simulink model "electrolyser_v4"  (R2022a)
settings: Solver=VariableStepAuto  StartTime=0.0  StopTime=10.0  RelTol=1e-3
model workspace: external: MATLAB File parameters_SS.m (data not in the file)
undefined symbols (not defined in the file or in its folder): clnt, const, input, pemel
libraries: fl_lib x24, nesl_utility x6, SimscapeFluids_lib x3
(part 2 of 2)

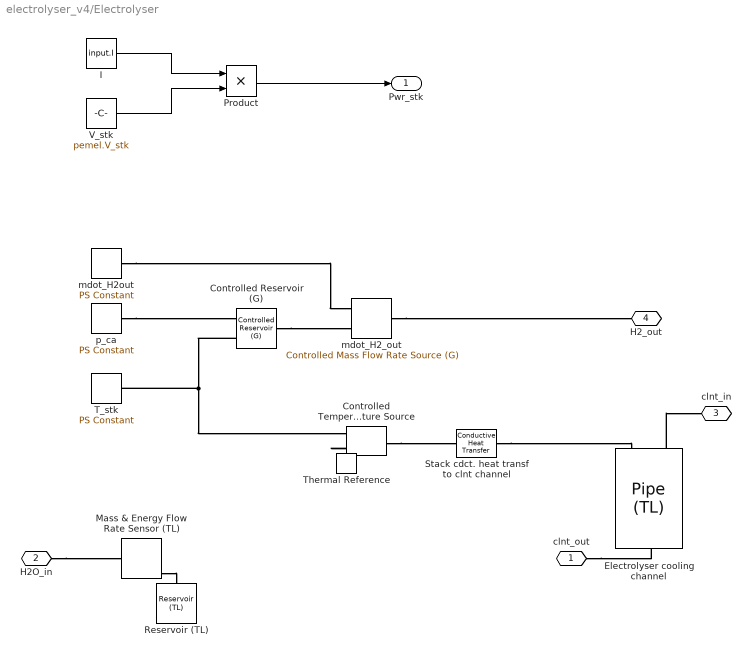
== system electrolyser_v4/Electrolyser ==
  Controlled Temperature Source : fl_lib/Thermal/Thermal Sources/Controlled Temperature Source
      settings: SourceProductBaseCode=PW,SS,VE
  Controlled Reservoir (G) : fl_lib/Gas/Elements/Controlled Reservoir (G)  area_A=pemel.totAc_ch_stk m^2
      settings: SourceProductBaseCode=PW,SS,VE  InternalSimscapePortConfiguration="{\"Bottom\":[],\"Left\":[{\"id\":\"A\",\"label\":\"A\",\"type\":\"foundation.gas.gas\"}],\"Right\":[{\"id\":\"T_in\",\"label\":\"T\",\"type\":\"input\"},{\"id\":\"p_in\",\"label\":\"P\",\"type\":\"input\"}],\"Top\":[]}"
  Electrolyser cooling channel : SimscapeFluids_lib/Thermal Liquid/Pipes & Fittings/Pipe (TL)  dynamic_compressibility=simscape.enum.onoff.off  inertia=simscape.enum.onoff.off  num_segments=1  pipe_length=pemel.L_clt m  area=pemel.totAc_clt_stk m^2  wall_spec=fluids.thermal_liquid.pipes_fittings.enum.wall_spec.rigid  Dh=pemel.Dh_clt m  wall_compliance=1.2e-6 m/MPa  wall_time_constant=0.01 s  elevation_spec=foundation.enum.constant_variable.constant  elevation_gain=0 m  g=9.81 m/s^2  pressure_loss_spec=fluids.thermal_liquid.pipes_fittings.enum.PressureLossSpec.Nominal  local_pressure_loss_spec=fluids.thermal_liquid.pipes_fittings.enum.LocalLossSpec.AggregateLength  length_add=1 m  loss_coefficient=0.1  roughness=15e-6 m  Re_friction_TLU=[400, 1000, 1500, 3000, 4000, 6000, 10000, 20000, 40000, 60000, 100000, 100000000]  friction_factor_TLU=[.264, .112, .071, .0417, .0387, .0268, .025, .0232, .0226, .022, .0214, .0214]  shape_factor=64  Re_lam=100000000  Re_tur=100000001  mdot_nominal=clnt.mdot_stk kg/s  p_diff_nominal=clnt.dp_stk Pa  mdot_threshold=1e-12 kg/s  heat_transfer_spec=fluids.thermal_liquid.pipes_fittings.enum.HeatTransferSpec.Nominal  mdot_nominal_heat=clnt.mdot_stk kg/s  T_in_nominal=clnt.T_stk_in K  T_out_nominal=clnt.T_stk_in + clnt.dT_stk K  p_in_nominal_heat=clnt.p_stk_in Pa  T_wall_nominal=pemel.T_stk K  a_coeff=0.023  b_Re_power=0.8  c_Pr_power=0.4  Nu_lam=3.66  Re_Colburn_TLU=[100, 150, 1000]  Colburn_factor_TLU=[.019, .013, .002]  Re_Nu_TLU=[100, 150, 1000]  Pr_Nu_TLU=[1, 10]  Nu_TLU=[3.72, 4.21; 3.75, 4.44; 4.21, 7.15]  T0_vec=amb.T K  p0_vec=0.101325 MPa  mdot0=0.1 kg/s
      settings: SourceProductBaseCode=SH
  I : Constant  Value=input.I
  Mass & Energy Flow Rate Sensor (TL) : fl_lib/Thermal Liquid/Sensors/Mass & Energy Flow Rate Sensor (TL)
      settings: SourceProductBaseCode=PW,SS,VE  InternalSimscapePortConfiguration="{\"Bottom\":[],\"Left\":[{\"id\":\"A\",\"label\":\"A\",\"type\":\"foundation.thermal_liquid.thermal_liquid\"}],\"Right\":[{\"id\":\"B\",\"label\":\"B\",\"type\":\"foundation.thermal_liquid.thermal_liquid\"},{\"id\":\"M\",\"label\":\"M\",\"type\":\"output\"},{\"id\":\"PHI\",\"label\":\"Phi\",\"type\":\"output\"}],\"Top\":[]}"
  Product : Product
  Reservoir (TL) : fl_lib/Thermal Liquid/Elements/Reservoir (TL)  pressure_spec=foundation.enum.pressure_spec.atmospheric  reservoir_pressure=0.101325 MPa  reservoir_temperature=293.15 K  area=pemel.totAc_ch_stk m^2
      settings: SourceProductBaseCode=PW,SS,VE
  Stack cdct. heat transf to clnt channel : fl_lib/Thermal/Thermal Elements/Conductive Heat Transfer  area=pemel.Prm_clt*pemel.L_clt m^2  thickness=pemel.thk_bp m  th_cond=pemel.k_bp W/(m*K)  T_specify=off  T_priority=None  T=0 K  T_nominal_specify=off  T_nominal_unit=K  T_nominal_value=1  Q_specify=off  Q_priority=None  Q=0 W  Q_nominal_specify=off  Q_nominal_unit=W  Q_nominal_value=1
      settings: SourceProductBaseCode=PW,SS,VE
  T_stk : fl_lib/Physical Signals/Sources/PS Constant  constant=353
      settings: SourceProductBaseCode=PW,SS,VE
  Thermal Reference : fl_lib/Thermal/Thermal Elements/Thermal Reference
      settings: SourceProductBaseCode=PW,SS,VE
  V_stk : Constant  Value=pemel.V_stk
  mdot_H2_out : fl_lib/Gas/Sources/Controlled Mass Flow Rate Source (G)  power_spec=foundation.enum.power_spec.none  area_A=pemel.Ac_ch m^2  area_B=pemel.Ac_ch m^2
      settings: SourceProductBaseCode=PW,SS,VE  InternalSimscapePortConfiguration="{\"Bottom\":[],\"Left\":[{\"id\":\"A\",\"label\":\"A\",\"type\":\"foundation.gas.gas\"},{\"id\":\"M\",\"label\":\"M\",\"type\":\"input\"}],\"Right\":[{\"id\":\"B\",\"label\":\"B\",\"type\":\"foundation.gas.gas\"}],\"Top\":[]}"
  mdot_H2out : fl_lib/Physical Signals/Sources/PS Constant  constant=h2.mdot_stk kg/s
      settings: SourceProductBaseCode=PW,SS,VE
  p_ca : fl_lib/Physical Signals/Sources/PS Constant  constant=pemel.p_ca Pa
      settings: SourceProductBaseCode=PW,SS,VE
  clnt_out : PMIOPort  Side=Left
  H2O_in : PMIOPort  Port=2  Side=Left
  clnt_in : PMIOPort  Port=3  Side=Right
  H2_out : PMIOPort  Port=4  Side=Right
  Pwr_stk : Outport
  wires:
  I/1 -> Product/1
  V_stk/1 -> Product/2
  Product/1 -> Pwr_stk/1
  connections:
  mdot_H2_out/RConn1 -- H2_out/RConn1
  H2O_in/RConn1 -- Mass & Energy Flow Rate Sensor (TL)/LConn1
  Controlled Reservoir (G)/RConn1 -- Controlled Temperature Source/RConn1 -- T_stk/RConn1
  Controlled Reservoir (G)/LConn1 -- mdot_H2_out/LConn1
  p_ca/RConn1 -- Controlled Reservoir (G)/RConn2
  Mass & Energy Flow Rate Sensor (TL)/RConn1 -- Reservoir (TL)/LConn1
  Stack cdct. heat transf to clnt channel/RConn1 -- Electrolyser cooling channel/LConn2
  clnt_out/RConn1 -- Electrolyser cooling channel/RConn1
  Controlled Temperature Source/LConn1 -- Stack cdct. heat transf to clnt channel/LConn1
  Electrolyser cooling channel/LConn1 -- clnt_in/RConn1
  Controlled Temperature Source/RConn2 -- Thermal Reference/LConn1
  mdot_H2out/RConn1 -- mdot_H2_out/LConn2
